simulink model "matrixOps"  (R2024b)
settings: Solver=VariableStepAuto  StartTime=0.0  StopTime=10.0  RelTol=1e-3
values from neighbouring files (symbols this model uses):
  d = [1 2 4 5]    [matrixOpsVar.mat]
  m1 = [1  2; 3  4; 5  6]    [matrixOpsVar.mat]
  m2 = [1  1  1; 1  1  1]    [matrixOpsVar.mat]
  X = [1  2  3  4; 5  6  7  8; 9  10  11  21]    [matrixOpsVar.mat]
undefined symbols (not defined in the file or in its folder): gcbh
libraries: matrix_library x6
settings Model: Creator=optimus  LastModifiedBy=optimus

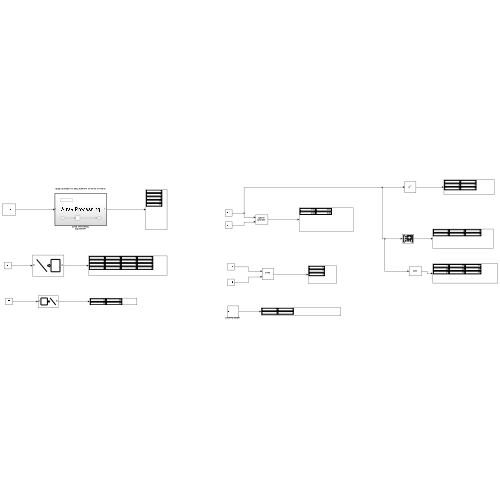
[thumbnail: Simulink's stored preview of the top-level diagram]
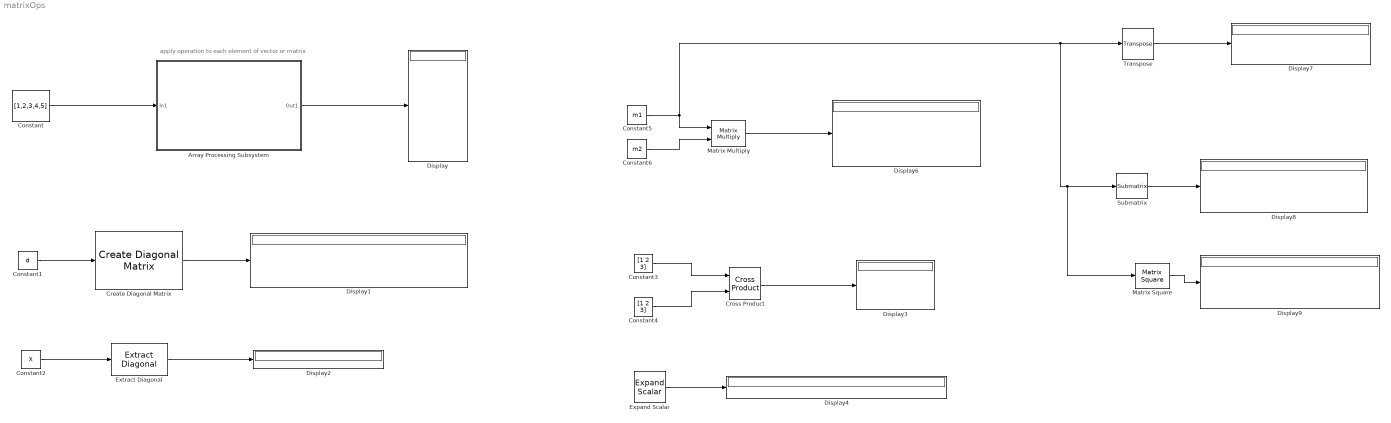
== system matrixOps ==
  note: apply operation to each element of vector or matrix
  Array Processing Subsystem : Subsystem  ClipboardFcn=set_param(gcbh,'LinkStatus','breakWithoutHierarchy'); set_param(gcbh,'Mask','off'); set_param(gcbh,'MaskType',''); set_param(gcbh,'MaskDescription',''); set_param(gcbh,'OpenFcn',''); set_param(gcbh,'CopyFcn','')  TreatAsAtomicUnit=on
  Constant : Constant  Value=[1,2,3,4,5]
  Constant1 : Constant  Value=d
  Constant2 : Constant  Value=X  VectorParams1D=off
  Constant3 : Constant  Value=[1 2 3]  VectorParams1D=off
  Constant4 : Constant  Value=[1 2 3]
  Constant5 : Constant  Value=m1
  Constant6 : Constant  Value=m2
  Create Diagonal Matrix : matrix_library/Create Diagonal Matrix
      settings: LibrarySourceBlock=|
      | simulink/Matrix
      | Operations/Create Diagonal
      | Matrix
  Cross Product : matrix_library/Cross Product
  Display{,1..4,6..9} (9 alike) : Display
  Expand Scalar : ExpandScalar  OutputDimensions=[2 2]
  Extract Diagonal : matrix_library/Extract Diagonal
      settings: LibrarySourceBlock=|
      | simulink/Matrix
      | Operations/Extract Diagonal
  Matrix Square : matrix_library/Matrix Square  OutMin=[]  OutMax=[]
      settings: LibrarySourceBlock=|
      | simulink/Matrix
      | Operations/Matrix
      | Square
  Matrix Multiply : Product  Multiplication=Matrix(*)
  Submatrix : matrix_library/Submatrix  RowSpan=All rows  RowStartMode=First  RowStartIndex=1  RowEndMode=Last  RowEndIndex=1  ColSpan=Range of columns  ColStartMode=First  ColStartIndex=1  ColEndMode=Offset from last  ColEndIndex=0
  Transpose : matrix_library/Transpose
  wires:
  Constant/1 -> Array Processing Subsystem/1(In1)
  Array Processing Subsystem/1(Out1) -> Display/1
  Create Diagonal Matrix/1 -> Display1/1
  Constant1/1 -> Create Diagonal Matrix/1
  Constant2/1 -> Extract Diagonal/1
  Extract Diagonal/1 -> Display2/1
  Cross Product/1 -> Display3/1
  Constant3/1 -> Cross Product/1
  Constant4/1 -> Cross Product/2
  Expand Scalar/1 -> Display4/1
  Matrix Multiply/1 -> Display6/1
  Transpose/1 -> Display7/1
  Submatrix/1 -> Display8/1
  Matrix Square/1 -> Display9/1
  Constant6/1 -> Matrix Multiply/2
  Constant5/1 -> Matrix Square/1, Submatrix/1, Transpose/1, Matrix Multiply/1

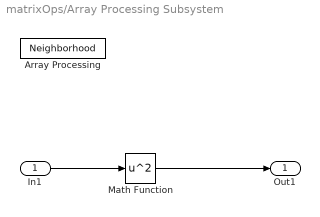
== system matrixOps/Array Processing Subsystem ==
  In1 : Inport
  Array Processing : Neighborhood  UsageType=ArrayFun
  Math Function : Math  Operator=square
  Out1 : Outport  ConcatenationDimension=[1 2]
  wires:
  In1/1 -> Math Function/1
  Math Function/1 -> Out1/1
